simulink model "HEV_Simu_V1_1_VectVir"  (R2018a)
settings: Solver=ode23s  StartTime=0.0  StopTime=660  FixedStep=0.001  EnableMultiTasking=on
PreLoadFcn:
  | HevSimuVccWs_V1_PreLoad
StartFcn:
  | tic
StopFcn:
  | toc
  | disp(['実時間の' num2str(max(tout)/toc) '倍速'])
model workspace (MAT data in the model file):
  Var = 0
undefined symbols (not defined in the file or in its folder): canChannel
libraries: canmsglib x55, canlib x35, simulink x2, sldrtlib x1
(part 4 of 4)

== system HEV_Simu_V1_1_VectVir/Controller/CtrlStrct_VNT_Level_2/VNT_Level_2_CAN/Gateway/Gateway PwtrCAN/Gateway_VehCAN_Receive_50ms ==
  VehCAN_Msg : Inport
  function : TriggerPort  TriggerType=function-call  VariantControl=Variant
  Gateway_VehCAN Unpack2 : canmsglib/CAN Unpack  CANdbFile=HEV_CANDB.dbc  MsgList=BodyCtrl_VehCAN_Tx  MsgName=BodyCtrl_VehCAN_Tx  MsgIDType=Extended (29-bit identifier)  MsgIdentifier=218079272  MsgLength=8  SignalInfo=BdyCtrl_Door_open_flag$1$1$1$2$1$0$1$0$0$1$#BdyCtrl_Engine_hood_open_flag$1$1$1$2$1$0$1$0$0$1$#BdyCtrl_Idlestop_cancel$0$1$1$2$1$0$1$0$0$1$#  NSignals=3  IDPort=off  TimestampPort=off  ErrorPort=off  RemotePort=off  LengthPort=off  StatusPort=off  StartBits=str2num('[int32(1);int32(1);int32(0)]')  SignalSizes=str2num('[int32(1);int32(1);int32(1)]')  ByteOrders=str2num('[int32(1);int32(1);int32(1)]')  DataTypes=str2num('[int32(2);int32(2);int32(2)]')  MultiplexTypes=str2num('[int32(1);int32(1);int32(1)]')  MultiplexValues=str2num('[double(0);double(0);double(0)]')  Factors=str2num('[double(1);double(1);double(1)]')  Offsets=str2num('[double(0);double(0);double(0)]')  Minimums=str2num('[double(0);double(0);double(0)]')  Maximums=str2num('[double(1);double(1);double(1)]')  ApplyMinMax=off
      settings: AttributesFormatString=<CANdbFile = %<CANdbFile>>  SourceProductName=Simulink Real-Time  SourceProductBaseCode=XP  DataFormat=CANdb specified signals
  Gateway_VehCAN Unpack4 : canmsglib/CAN Unpack  CANdbFile=HEV_CANDB.dbc  MsgList=HVAC_Ctrl_VehCAN_Tx  MsgName=HVAC_Ctrl_VehCAN_Tx  MsgIDType=Extended (29-bit identifier)  MsgIdentifier=218095751  MsgLength=8  SignalInfo=HVAC_Ctrl_Idlestop_cancel$1$1$1$2$1$0$1$0$0$1$#HVAC_Ctrl_Idlestop_enbl$0$1$1$2$1$0$1$0$0$1$#  NSignals=2  IDPort=off  TimestampPort=off  ErrorPort=off  RemotePort=off  LengthPort=off  StatusPort=off  StartBits=str2num('[int32(1);int32(0)]')  SignalSizes=str2num('[int32(1);int32(1)]')  ByteOrders=str2num('[int32(1);int32(1)]')  DataTypes=str2num('[int32(2);int32(2)]')  MultiplexTypes=str2num('[int32(1);int32(1)]')  MultiplexValues=str2num('[double(0);double(0)]')  Factors=str2num('[double(1);double(1)]')  Offsets=str2num('[double(0);double(0)]')  Minimums=str2num('[double(0);double(0)]')  Maximums=str2num('[double(1);double(1)]')  ApplyMinMax=off
      settings: AttributesFormatString=<CANdbFile = %<CANdbFile>>  SourceProductName=Simulink Real-Time  SourceProductBaseCode=XP  DataFormat=CANdb specified signals
  Gateway_VehCAN Unpack5 : canmsglib/CAN Unpack  CANdbFile=HEV_CANDB.dbc  MsgList=SteerCtrl_VehCAN_Tx  MsgName=SteerCtrl_VehCAN_Tx  MsgIDType=Extended (29-bit identifier)  MsgIdentifier=218066963  MsgLength=8  SignalInfo=StrgCtrl_Steer_angle$0$16$1$1$1$0$3.125000e-02$0$-720$720$#  NSignals=1  IDPort=off  TimestampPort=off  ErrorPort=off  RemotePort=off  LengthPort=off  StatusPort=off  StartBits=str2num('[int32(0)]')  SignalSizes=str2num('[int32(16)]')  ByteOrders=str2num('[int32(1)]')  DataTypes=str2num('[int32(1)]')  MultiplexTypes=str2num('[int32(1)]')  MultiplexValues=str2num('[double(0)]')  Factors=str2num('[double(3.125000e-02)]')  Offsets=str2num('[double(0)]')  Minimums=str2num('[double(-720)]')  Maximums=str2num('[double(720)]')  ApplyMinMax=off
      settings: AttributesFormatString=<CANdbFile = %<CANdbFile>>  SourceProductName=Simulink Real-Time  SourceProductBaseCode=XP  DataFormat=CANdb specified signals
  BdyCtrl_Door_open_flag : Outport
  BdyCtrl_Engine_hood_open_flag : Outport  Port=2
  BdyCtrl_Idlestop_cancel : Outport  Port=3
  HVAC_Ctrl_Idlestop_cancel : Outport  Port=4
  HVAC_Ctrl_Idlestop_enbl : Outport  Port=5
  StrgCtrl_Steer_angle : Outport  Port=6
  wires:
  Gateway_VehCAN Unpack5/1 -> StrgCtrl_Steer_angle/1  "VehCAN_StrgCtrl_Steer_angle"
  VehCAN_Msg/1 -> Gateway_VehCAN Unpack5/1, Gateway_VehCAN Unpack4/1, Gateway_VehCAN Unpack2/1
  Gateway_VehCAN Unpack4/1 -> HVAC_Ctrl_Idlestop_cancel/1  "VehCAN_HVAC_Ctrl_Idlestop_cancel"
  Gateway_VehCAN Unpack4/2 -> HVAC_Ctrl_Idlestop_enbl/1  "VehCAN_HVAC_Ctrl_Idlestop_enbl"
  Gateway_VehCAN Unpack2/1 -> BdyCtrl_Door_open_flag/1  "VehCAN_BdyCtrl_Door_open_flag"
  Gateway_VehCAN Unpack2/3 -> BdyCtrl_Idlestop_cancel/1  "VehCAN_BdyCtrl_Idlestop_cancel"
  Gateway_VehCAN Unpack2/2 -> BdyCtrl_Engine_hood_open_flag/1  "VehCAN_BdyCtrl_Engine_hood_open_flag"

== system HEV_Simu_V1_1_VectVir/Controller/CtrlStrct_VNT_Level_2/VNT_Level_2_CAN/Gateway/Gateway VehCAN/Gateway_InfoCAN_Receive_100ms ==
  InfoCAN_Msg : Inport
  function : TriggerPort  TriggerType=function-call  VariantControl=Variant
  Radar_InfoCAN Unpack : canmsglib/CAN Unpack  CANdbFile=HEV_CANDB.dbc  MsgList=Radar_InfoCAN_Tx  MsgName=Radar_InfoCAN_Tx  MsgIDType=Extended (29-bit identifier)  MsgIdentifier=218038400  MsgLength=8  SignalInfo=Radar_Relative_distance$0$16$1$2$1$0$1.000000e-02$0$0$500$#Radar_Relative_velocity$16$16$1$1$1$0$1.000000e-02$0$-50$50$#  NSignals=2  IDPort=off  TimestampPort=off  ErrorPort=off  RemotePort=off  LengthPort=off  StatusPort=off  StartBits=str2num('[int32(0);int32(16)]')  SignalSizes=str2num('[int32(16);int32(16)]')  ByteOrders=str2num('[int32(1);int32(1)]')  DataTypes=str2num('[int32(2);int32(1)]')  MultiplexTypes=str2num('[int32(1);int32(1)]')  MultiplexValues=str2num('[double(0);double(0)]')  Factors=str2num('[double(1.000000e-02);double(1.000000e-02)]')  Offsets=str2num('[double(0);double(0)]')  Minimums=str2num('[double(0);double(-50)]')  Maximums=str2num('[double(500);double(50)]')  ApplyMinMax=off
      settings: AttributesFormatString=<CANdbFile = %<CANdbFile>>  SourceProductName=Simulink Real-Time  SourceProductBaseCode=XP  DataFormat=CANdb specified signals
  Radar_Relative_distance : Outport
  Radar_Relative_velocity : Outport  Port=2
  wires:
  Radar_InfoCAN Unpack/2 -> Radar_Relative_velocity/1  "InfoCAN_Radar_Relative_velocity"
  InfoCAN_Msg/1 -> Radar_InfoCAN Unpack/1
  Radar_InfoCAN Unpack/1 -> Radar_Relative_distance/1  "InfoCAN_Radar_Relative_distance"

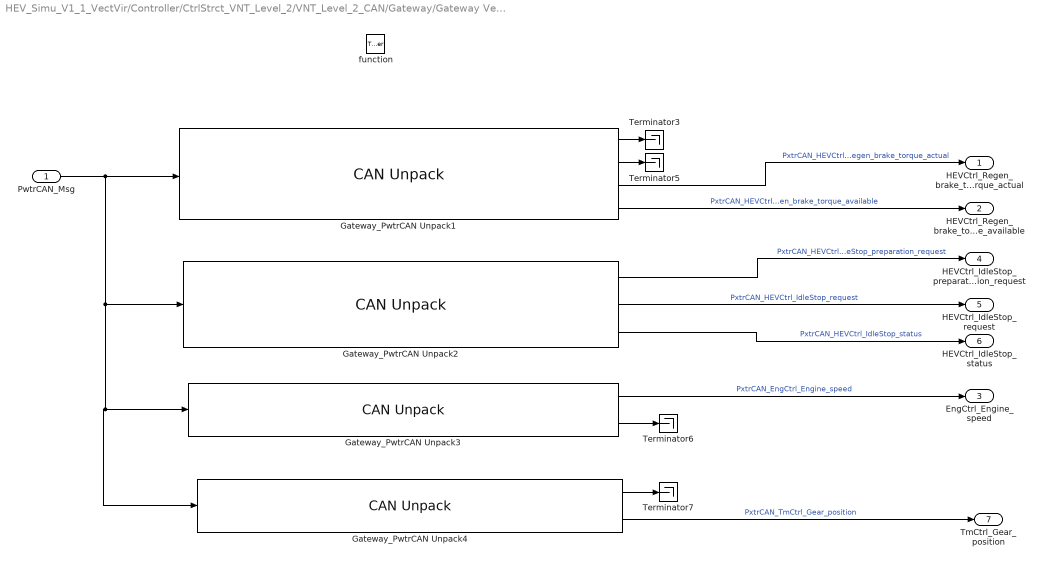
== system HEV_Simu_V1_1_VectVir/Controller/CtrlStrct_VNT_Level_2/VNT_Level_2_CAN/Gateway/Gateway VehCAN/Gateway_PwtrCAN_Receive_10ms ==
  PwtrCAN_Msg : Inport
  function : TriggerPort  TriggerType=function-call  VariantControl=Variant
  Gateway_PwtrCAN Unpack1 : canmsglib/CAN Unpack  CANdbFile=HEV_CANDB.dbc  MsgList=HEV_Ctrl_PwtrCAN_Tx_1  MsgName=HEV_Ctrl_PwtrCAN_Tx_1  MsgIDType=Extended (29-bit identifier)  MsgIdentifier=218046594  MsgLength=8  SignalInfo=HEVCtrl_Engine_torque_request$0$16$1$1$1$0$1.562500e-02$0$-300$300$#HEVCtrl_Motor_torque_request$16$16$1$1$1$0$1.562500e-02$0$-300$300$#HEVCtrl_Regen_brake_torque_actua$48$16$1$1$1$0$6.250000e-02$0$-300$3000$#HEVCtrl_Regen_brake_torque_avail$32$16$1$1$1$0$6.250000e-02$0$-300$3000$#  NSignals=4  IDPort=off  TimestampPort=off  ErrorPort=off  RemotePort=off  LengthPort=off  StatusPort=off  StartBits=str2num('[int32(0);int32(16);int32(48);int32(32)]')  SignalSizes=str2num('[int32(16);int32(16);int32(16);int32(16)]')  ByteOrders=str2num('[int32(1);int32(1);int32(1);int32(1)]')  DataTypes=str2num('[int32(1);int32(1);int32(1);int32(1)]')  MultiplexTypes=str2num('[int32(1);int32(1);int32(1);int32(1)]')  MultiplexValues=str2num('[double(0);double(0);double(0);double(0)]')  Factors=str2num('[double(1.562500e-02);double(1.562500e-02);double(6.250000e-02);double(6.250000e-02)]')  Offsets=str2num('[double(0);double(0);double(0);double(0)]')  Minimums=str2num('[double(-300);double(-300);double(-300);double(-300)]')  Maximums=str2num('[double(300);double(300);double(3000);double(3000)]')  ApplyMinMax=off
      settings: AttributesFormatString=<CANdbFile = %<CANdbFile>>  SourceProductName=Simulink Real-Time  SourceProductBaseCode=XP  DataFormat=CANdb specified signals
  Gateway_PwtrCAN Unpack2 : canmsglib/CAN Unpack  CANdbFile=HEV_CANDB.dbc  MsgList=HEV_Ctrl_PwtrCAN_Tx_2  MsgName=HEV_Ctrl_PwtrCAN_Tx_2  MsgIDType=Extended (29-bit identifier)  MsgIdentifier=218046850  MsgLength=8  SignalInfo=HEV_IdleStopCtrl_preparation_req$0$1$1$2$1$0$1$0$0$1$#HEV_IdleStopCtrl_request$1$1$1$2$1$0$1$0$0$1$#HEV_IdleStopCtrl_status$2$1$1$2$1$0$1$0$0$1$#  NSignals=3  IDPort=off  TimestampPort=off  ErrorPort=off  RemotePort=off  LengthPort=off  StatusPort=off  StartBits=str2num('[int32(0);int32(1);int32(2)]')  SignalSizes=str2num('[int32(1);int32(1);int32(1)]')  ByteOrders=str2num('[int32(1);int32(1);int32(1)]')  DataTypes=str2num('[int32(2);int32(2);int32(2)]')  MultiplexTypes=str2num('[int32(1);int32(1);int32(1)]')  MultiplexValues=str2num('[double(0);double(0);double(0)]')  Factors=str2num('[double(1);double(1);double(1)]')  Offsets=str2num('[double(0);double(0);double(0)]')  Minimums=str2num('[double(0);double(0);double(0)]')  Maximums=str2num('[double(1);double(1);double(1)]')  ApplyMinMax=off
      settings: AttributesFormatString=<CANdbFile = %<CANdbFile>>  SourceProductName=Simulink Real-Time  SourceProductBaseCode=XP  DataFormat=CANdb specified signals
  Gateway_PwtrCAN Unpack3 : canmsglib/CAN Unpack  CANdbFile=HEV_CANDB.dbc  MsgList=EngineCtrl_PwtrCAN_Tx  MsgName=EngineCtrl_PwtrCAN_Tx  MsgIDType=Extended (29-bit identifier)  MsgIdentifier=218050560  MsgLength=8  SignalInfo=EngCtrl_Engine_speed$0$16$1$2$1$0$1.250000e-01$0$0$8192$#EngCtrl_Engine_torque_actual$16$16$1$1$1$0$1.562500e-02$0$-300$300$#  NSignals=2  IDPort=off  TimestampPort=off  ErrorPort=off  RemotePort=off  LengthPort=off  StatusPort=off  StartBits=str2num('[int32(0);int32(16)]')  SignalSizes=str2num('[int32(16);int32(16)]')  ByteOrders=str2num('[int32(1);int32(1)]')  DataTypes=str2num('[int32(2);int32(1)]')  MultiplexTypes=str2num('[int32(1);int32(1)]')  MultiplexValues=str2num('[double(0);double(0)]')  Factors=str2num('[double(1.250000e-01);double(1.562500e-02)]')  Offsets=str2num('[double(0);double(0)]')  Minimums=str2num('[double(0);double(-300)]')  Maximums=str2num('[double(8192);double(300)]')  ApplyMinMax=off
      settings: AttributesFormatString=<CANdbFile = %<CANdbFile>>  SourceProductName=Simulink Real-Time  SourceProductBaseCode=XP  DataFormat=CANdb specified signals
  Gateway_PwtrCAN Unpack4 : canmsglib/CAN Unpack  CANdbFile=HEV_CANDB.dbc  MsgList=TransmCtrl_PwtrCAN_Tx  MsgName=TransmCtrl_PwtrCAN_Tx  MsgIDType=Extended (29-bit identifier)  MsgIdentifier=218054659  MsgLength=8  SignalInfo=TmCtrl_Clutch_position$0$8$1$2$1$0$1.000000e-02$0$0$1$#TmCtrl_Gear_position$8$8$1$2$1$0$1$0$0$5$#  NSignals=2  IDPort=off  TimestampPort=off  ErrorPort=off  RemotePort=off  LengthPort=off  StatusPort=off  StartBits=str2num('[int32(0);int32(8)]')  SignalSizes=str2num('[int32(8);int32(8)]')  ByteOrders=str2num('[int32(1);int32(1)]')  DataTypes=str2num('[int32(2);int32(2)]')  MultiplexTypes=str2num('[int32(1);int32(1)]')  MultiplexValues=str2num('[double(0);double(0)]')  Factors=str2num('[double(1.000000e-02);double(1)]')  Offsets=str2num('[double(0);double(0)]')  Minimums=str2num('[double(0);double(0)]')  Maximums=str2num('[double(1);double(5)]')  ApplyMinMax=off
      settings: AttributesFormatString=<CANdbFile = %<CANdbFile>>  SourceProductName=Simulink Real-Time  SourceProductBaseCode=XP  DataFormat=CANdb specified signals
  Terminator{3,5..7} (4 alike) : Terminator
  HEVCtrl_Regen_brake_torque_actual : Outport
  HEVCtrl_Regen_brake_torque_available : Outport  Port=2
  EngCtrl_Engine_speed : Outport  Port=3
  HEVCtrl_IdleStop_preparation_request : Outport  Port=4
  HEVCtrl_IdleStop_request : Outport  Port=5
  HEVCtrl_IdleStop_status : Outport  Port=6
  TmCtrl_Gear_position : Outport  Port=7
  wires:
  Gateway_PwtrCAN Unpack1/4 -> HEVCtrl_Regen_brake_torque_available/1  "PxtrCAN_HEVCtrl_Regen_brake_torque_available"
  Gateway_PwtrCAN Unpack2/1 -> HEVCtrl_IdleStop_preparation_request/1  "PxtrCAN_HEVCtrl_IdleStop_preparation_request"
  Gateway_PwtrCAN Unpack3/1 -> EngCtrl_Engine_speed/1  "PxtrCAN_EngCtrl_Engine_speed"
  Gateway_PwtrCAN Unpack3/2 -> Terminator6/1
  Gateway_PwtrCAN Unpack1/2 -> Terminator5/1
  Gateway_PwtrCAN Unpack1/1 -> Terminator3/1
  Gateway_PwtrCAN Unpack4/2 -> TmCtrl_Gear_position/1  "PxtrCAN_TmCtrl_Gear_position"
  PwtrCAN_Msg/1 -> Gateway_PwtrCAN Unpack1/1, Gateway_PwtrCAN Unpack3/1, Gateway_PwtrCAN Unpack4/1, Gateway_PwtrCAN Unpack2/1
  Gateway_PwtrCAN Unpack2/2 -> HEVCtrl_IdleStop_request/1  "PxtrCAN_HEVCtrl_IdleStop_request"
  Gateway_PwtrCAN Unpack4/1 -> Terminator7/1
  Gateway_PwtrCAN Unpack1/3 -> HEVCtrl_Regen_brake_torque_actual/1  "PxtrCAN_HEVCtrl_Regen_brake_torque_actual"
  Gateway_PwtrCAN Unpack2/3 -> HEVCtrl_IdleStop_status/1  "PxtrCAN_HEVCtrl_IdleStop_status"

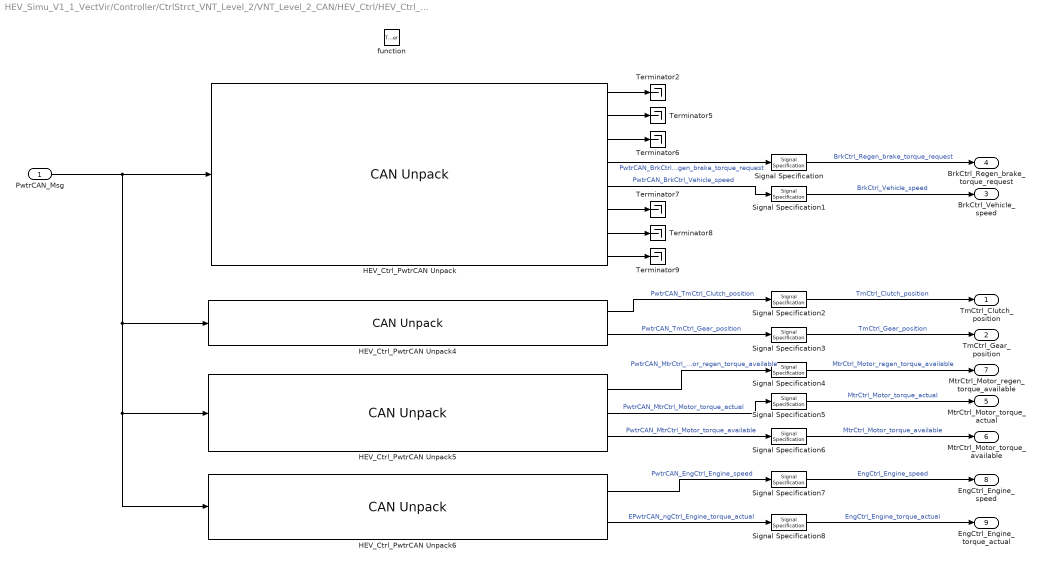
== system HEV_Simu_V1_1_VectVir/Controller/CtrlStrct_VNT_Level_2/VNT_Level_2_CAN/HEV_Ctrl/HEV_Ctrl_PwtrCAN_Rx/HEV_Ctrl_PwtrCAN_Receive_10ms ==
  PwtrCAN_Msg : Inport
  function : TriggerPort  TriggerType=function-call  VariantControl=Variant
  HEV_Ctrl_PwtrCAN Unpack : canmsglib/CAN Unpack  CANdbFile=HEV_CANDB.dbc  MsgList=Gateway_PwtrCAN_Tx_2  MsgName=Gateway_PwtrCAN_Tx_2  MsgIDType=Extended (29-bit identifier)  MsgIdentifier=218088325  MsgLength=8  SignalInfo=BdyCtrl_Door_open_flag_G$60$1$1$2$1$0$1$0$0$1$#BdyCtrl_Engine_hood_open_flg_G$59$1$1$2$1$0$1$0$0$1$#BdyCtrl_Idlestop_cancel_G$58$1$1$2$1$0$1$0$0$1$#BrkCtrl_Regen_brake_torque_re_G$16$16$1$1$1$0$1.000000e-02$0$-300$300$#BrkCtrl_Vehicle_speed_G$0$16$1$2$1$0$1.000000e-01$0$0$180$#HVAC_Ctrl_Idlestop_cancel_G$57$1$1$2$1$0$1$0$0$1$#HVAC_Ctrl_Idlestop_enbl_G$56$1$1$2$1$0$1$0$0$1$#StrgCtrl_Steer_angle_G$32$16$1$1$1$0$3.125000e-02$0$-720$720$#  NSignals=8  IDPort=off  TimestampPort=off  ErrorPort=off  RemotePort=off  LengthPort=off  StatusPort=off  StartBits=str2num('[int32(60);int32(59);int32(58);int32(16);int32(0);int32(57);int32(56);int32(32)]')  SignalSizes=str2num('[int32(1);int32(1);int32(1);int32(16);int32(16);int32(1);int32(1);int32(16)]')  ByteOrders=str2num('[int32(1);int32(1);int32(1);int32(1);int32(1);int32(1);int32(1);int32(1)]')  DataTypes=str2num('[int32(2);int32(2);int32(2);int32(1);int32(2);int32(2);int32(2);int32(1)]')  MultiplexTypes=str2num('[int32(1);int32(1);int32(1);int32(1);int32(1);int32(1);int32(1);int32(1)]')  MultiplexValues=str2num('[double(0);double(0);double(0);double(0);double(0);double(0);double(0);double(0)]')  Factors=str2num('[double(1);double(1);double(1);double(1.000000e-02);double(1.000000e-01);double(1);double(1);double(3.125000e-02)]')  Offsets=str2num('[double(0);double(0);double(0);double(0);double(0);double(0);double(0);double(0)]')  Minimums=str2num('[double(0);double(0);double(0);double(-300);double(0);double(0);double(0);double(-720)]')  Maximums=str2num('[double(1);double(1);double(1);double(300);double(180);double(1);double(1);double(720)]')  ApplyMinMax=off
      settings: AttributesFormatString=<CANdbFile = %<CANdbFile>>  SourceProductName=Simulink Real-Time  SourceProductBaseCode=XP  DataFormat=CANdb specified signals
  HEV_Ctrl_PwtrCAN Unpack4 : canmsglib/CAN Unpack  CANdbFile=HEV_CANDB.dbc  MsgList=TransmCtrl_PwtrCAN_Tx  MsgName=TransmCtrl_PwtrCAN_Tx  MsgIDType=Extended (29-bit identifier)  MsgIdentifier=218054659  MsgLength=8  SignalInfo=TmCtrl_Clutch_position$0$8$1$2$1$0$1.000000e-02$0$0$1$#TmCtrl_Gear_position$8$8$1$2$1$0$1$0$0$5$#  NSignals=2  IDPort=off  TimestampPort=off  ErrorPort=off  RemotePort=off  LengthPort=off  StatusPort=off  StartBits=str2num('[int32(0);int32(8)]')  SignalSizes=str2num('[int32(8);int32(8)]')  ByteOrders=str2num('[int32(1);int32(1)]')  DataTypes=str2num('[int32(2);int32(2)]')  MultiplexTypes=str2num('[int32(1);int32(1)]')  MultiplexValues=str2num('[double(0);double(0)]')  Factors=str2num('[double(1.000000e-02);double(1)]')  Offsets=str2num('[double(0);double(0)]')  Minimums=str2num('[double(0);double(0)]')  Maximums=str2num('[double(1);double(5)]')  ApplyMinMax=off
      settings: AttributesFormatString=<CANdbFile = %<CANdbFile>>  SourceProductName=Simulink Real-Time  SourceProductBaseCode=XP  DataFormat=CANdb specified signals
  HEV_Ctrl_PwtrCAN Unpack5 : canmsglib/CAN Unpack  CANdbFile=HEV_CANDB.dbc  MsgList=MotorCtrl_PwtrCAN_Tx  MsgName=MotorCtrl_PwtrCAN_Tx  MsgIDType=Extended (29-bit identifier)  MsgIdentifier=218058883  MsgLength=8  SignalInfo=MtrCtrl_Motor_regen_torque_avail$32$16$1$1$1$0$1.000000e-02$0$-300$300$#MtrCtrl_Motor_torque_actual$0$16$1$1$1$0$1.000000e-02$0$-300$300$#MtrCtrl_Motor_torque_available$16$16$1$1$1$0$1.000000e-02$0$-300$300$#  NSignals=3  IDPort=off  TimestampPort=off  ErrorPort=off  RemotePort=off  LengthPort=off  StatusPort=off  StartBits=str2num('[int32(32);int32(0);int32(16)]')  SignalSizes=str2num('[int32(16);int32(16);int32(16)]')  ByteOrders=str2num('[int32(1);int32(1);int32(1)]')  DataTypes=str2num('[int32(1);int32(1);int32(1)]')  MultiplexTypes=str2num('[int32(1);int32(1);int32(1)]')  MultiplexValues=str2num('[double(0);double(0);double(0)]')  Factors=str2num('[double(1.000000e-02);double(1.000000e-02);double(1.000000e-02)]')  Offsets=str2num('[double(0);double(0);double(0)]')  Minimums=str2num('[double(-300);double(-300);double(-300)]')  Maximums=str2num('[double(300);double(300);double(300)]')  ApplyMinMax=off
      settings: AttributesFormatString=<CANdbFile = %<CANdbFile>>  SourceProductName=Simulink Real-Time  SourceProductBaseCode=XP  DataFormat=CANdb specified signals
  HEV_Ctrl_PwtrCAN Unpack6 : canmsglib/CAN Unpack  CANdbFile=HEV_CANDB.dbc  MsgList=EngineCtrl_PwtrCAN_Tx  MsgName=EngineCtrl_PwtrCAN_Tx  MsgIDType=Extended (29-bit identifier)  MsgIdentifier=218050560  MsgLength=8  SignalInfo=EngCtrl_Engine_speed$0$16$1$2$1$0$1.250000e-01$0$0$8192$#EngCtrl_Engine_torque_actual$16$16$1$1$1$0$1.562500e-02$0$-300$300$#  NSignals=2  IDPort=off  TimestampPort=off  ErrorPort=off  RemotePort=off  LengthPort=off  StatusPort=off  StartBits=str2num('[int32(0);int32(16)]')  SignalSizes=str2num('[int32(16);int32(16)]')  ByteOrders=str2num('[int32(1);int32(1)]')  DataTypes=str2num('[int32(2);int32(1)]')  MultiplexTypes=str2num('[int32(1);int32(1)]')  MultiplexValues=str2num('[double(0);double(0)]')  Factors=str2num('[double(1.250000e-01);double(1.562500e-02)]')  Offsets=str2num('[double(0);double(0)]')  Minimums=str2num('[double(0);double(-300)]')  Maximums=str2num('[double(8192);double(300)]')  ApplyMinMax=off
      settings: AttributesFormatString=<CANdbFile = %<CANdbFile>>  SourceProductName=Simulink Real-Time  SourceProductBaseCode=XP  DataFormat=CANdb specified signals
  Signal Specification{,1..8} (9 alike) : SignalSpecification
  Terminator{2,5..9} (6 alike) : Terminator
  TmCtrl_Clutch_position : Outport
  TmCtrl_Gear_position : Outport  Port=2
  BrkCtrl_Vehicle_speed : Outport  Port=3
  BrkCtrl_Regen_brake_torque_request : Outport  Port=4
  MtrCtrl_Motor_torque_actual : Outport  Port=5
  MtrCtrl_Motor_torque_available : Outport  Port=6
  MtrCtrl_Motor_regen_torque_available : Outport  Port=7
  EngCtrl_Engine_speed : Outport  Port=8
  EngCtrl_Engine_torque_actual : Outport  Port=9
  wires:
  HEV_Ctrl_PwtrCAN Unpack/1 -> Terminator2/1
  PwtrCAN_Msg/1 -> HEV_Ctrl_PwtrCAN Unpack4/1, HEV_Ctrl_PwtrCAN Unpack5/1, HEV_Ctrl_PwtrCAN Unpack6/1, HEV_Ctrl_PwtrCAN Unpack/1
  HEV_Ctrl_PwtrCAN Unpack/6 -> Terminator7/1
  HEV_Ctrl_PwtrCAN Unpack/3 -> Terminator6/1
  HEV_Ctrl_PwtrCAN Unpack/8 -> Terminator9/1
  HEV_Ctrl_PwtrCAN Unpack/5 -> Signal Specification1/1  "PwtrCAN_BrkCtrl_Vehicle_speed"
  HEV_Ctrl_PwtrCAN Unpack6/2 -> Signal Specification8/1  "EPwtrCAN_ngCtrl_Engine_torque_actual"
  HEV_Ctrl_PwtrCAN Unpack/2 -> Terminator5/1
  HEV_Ctrl_PwtrCAN Unpack/7 -> Terminator8/1
  HEV_Ctrl_PwtrCAN Unpack5/1 -> Signal Specification4/1  "PwtrCAN_MtrCtrl_Motor_regen_torque_available"
  HEV_Ctrl_PwtrCAN Unpack6/1 -> Signal Specification7/1  "PwtrCAN_EngCtrl_Engine_speed"
  HEV_Ctrl_PwtrCAN Unpack5/2 -> Signal Specification5/1  "PwtrCAN_MtrCtrl_Motor_torque_actual"
  HEV_Ctrl_PwtrCAN Unpack/4 -> Signal Specification/1  "PwtrCAN_BrkCtrl_Regen_brake_torque_request"
  HEV_Ctrl_PwtrCAN Unpack5/3 -> Signal Specification6/1  "PwtrCAN_MtrCtrl_Motor_torque_available"
  HEV_Ctrl_PwtrCAN Unpack4/1 -> Signal Specification2/1  "PwtrCAN_TmCtrl_Clutch_position"
  HEV_Ctrl_PwtrCAN Unpack4/2 -> Signal Specification3/1  "PwtrCAN_TmCtrl_Gear_position"
  Signal Specification/1 -> BrkCtrl_Regen_brake_torque_request/1  "BrkCtrl_Regen_brake_torque_request"
  Signal Specification1/1 -> BrkCtrl_Vehicle_speed/1  "BrkCtrl_Vehicle_speed"
  Signal Specification2/1 -> TmCtrl_Clutch_position/1  "TmCtrl_Clutch_position"
  Signal Specification3/1 -> TmCtrl_Gear_position/1  "TmCtrl_Gear_position"
  Signal Specification4/1 -> MtrCtrl_Motor_regen_torque_available/1  "MtrCtrl_Motor_regen_torque_available"
  Signal Specification5/1 -> MtrCtrl_Motor_torque_actual/1  "MtrCtrl_Motor_torque_actual"
  Signal Specification6/1 -> MtrCtrl_Motor_torque_available/1  "MtrCtrl_Motor_torque_available"
  Signal Specification7/1 -> EngCtrl_Engine_speed/1  "EngCtrl_Engine_speed"
  Signal Specification8/1 -> EngCtrl_Engine_torque_actual/1  "EngCtrl_Engine_torque_actual"

== system HEV_Simu_V1_1_VectVir/Controller/CtrlStrct_VNT_Level_2/VNT_Level_2_CAN/HEV_Ctrl/HEV_Ctrl_PwtrCAN_Rx/HEV_Ctrl_PwtrCAN_Receive_50ms ==
  PwtrCAN_Msg : Inport
  function : TriggerPort  TriggerType=function-call  VariantControl=Variant
  HEV_Ctrl_PwtrCAN Unpack2 : canmsglib/CAN Unpack  CANdbFile=HEV_CANDB.dbc  MsgList=Gateway_PwtrCAN_Tx_1  MsgName=Gateway_PwtrCAN_Tx_1  MsgIDType=Extended (29-bit identifier)  MsgIdentifier=218088069  MsgLength=8  SignalInfo=NAVI_Home_around_status_G$0$16$1$2$1$0$1$0$0$65535$#VMCtrl_PropTorqCmnd_G$24$16$1$1$1$0$1.000000e-02$0$-300$300$#VMCtrl_PropTorqStatus_G$16$8$1$2$1$0$1$0$0$7$#  NSignals=3  IDPort=off  TimestampPort=off  ErrorPort=off  RemotePort=off  LengthPort=off  StatusPort=off  StartBits=str2num('[int32(0);int32(24);int32(16)]')  SignalSizes=str2num('[int32(16);int32(16);int32(8)]')  ByteOrders=str2num('[int32(1);int32(1);int32(1)]')  DataTypes=str2num('[int32(2);int32(1);int32(2)]')  MultiplexTypes=str2num('[int32(1);int32(1);int32(1)]')  MultiplexValues=str2num('[double(0);double(0);double(0)]')  Factors=str2num('[double(1);double(1.000000e-02);double(1)]')  Offsets=str2num('[double(0);double(0);double(0)]')  Minimums=str2num('[double(0);double(-300);double(0)]')  Maximums=str2num('[double(65535);double(300);double(7)]')  ApplyMinMax=off
      settings: AttributesFormatString=<CANdbFile = %<CANdbFile>>  SourceProductName=Simulink Real-Time  SourceProductBaseCode=XP  DataFormat=CANdb specified signals
  HEV_Ctrl_PwtrCAN Unpack3 : canmsglib/CAN Unpack  CANdbFile=HEV_CANDB.dbc  MsgList=BatteryCtrl_PwtrCAN_Tx  MsgName=BatteryCtrl_PwtrCAN_Tx  MsgIDType=Extended (29-bit identifier)  MsgIdentifier=218071172  MsgLength=8  SignalInfo=BatCtrl_SOC$0$16$1$2$1$0$3.906250e-03$0$0$100$#  NSignals=1  IDPort=off  TimestampPort=off  ErrorPort=off  RemotePort=off  LengthPort=off  StatusPort=off  StartBits=str2num('[int32(0)]')  SignalSizes=str2num('[int32(16)]')  ByteOrders=str2num('[int32(1)]')  DataTypes=str2num('[int32(2)]')  MultiplexTypes=str2num('[int32(1)]')  MultiplexValues=str2num('[double(0)]')  Factors=str2num('[double(3.906250e-03)]')  Offsets=str2num('[double(0)]')  Minimums=str2num('[double(0)]')  Maximums=str2num('[double(100)]')  ApplyMinMax=off
      settings: AttributesFormatString=<CANdbFile = %<CANdbFile>>  SourceProductName=Simulink Real-Time  SourceProductBaseCode=XP  DataFormat=CANdb specified signals
  Signal Specification{,1..3} (4 alike) : SignalSpecification
  BatCtrl_SOC : Outport
  VMCtrl_PropTorqStatus : Outport  Port=2
  VMCtrl_PropTorqCmnd : Outport  Port=3
  NAVI_Home_around_status : Outport  Port=4
  wires:
  HEV_Ctrl_PwtrCAN Unpack2/1 -> Signal Specification/1  "PwtrCAN_NAVI_Home_around_status"
  PwtrCAN_Msg/1 -> HEV_Ctrl_PwtrCAN Unpack3/1, HEV_Ctrl_PwtrCAN Unpack2/1
  HEV_Ctrl_PwtrCAN Unpack3/1 -> Signal Specification3/1  "PwtrCAN_BatCtrl_SOC"
  HEV_Ctrl_PwtrCAN Unpack2/2 -> Signal Specification1/1  "PwtrCAN_VMCtrl_PropTorqCmnd"
  HEV_Ctrl_PwtrCAN Unpack2/3 -> Signal Specification2/1  "PwtrCAN_VMCtrl_PropTorqStatus"
  Signal Specification/1 -> NAVI_Home_around_status/1  "NAVI_Home_around_status"
  Signal Specification1/1 -> VMCtrl_PropTorqCmnd/1  "VMCtrl_PropTorqCmnd"
  Signal Specification2/1 -> VMCtrl_PropTorqStatus/1  "VMCtrl_PropTorqStatus"
  Signal Specification3/1 -> BatCtrl_SOC/1  "BatCtrl_SOC"

== system HEV_Simu_V1_1_VectVir/Controller/CtrlStrct_VNT_Level_2/VNT_Level_2_CAN/HVAC_Ctrl/HVAC_Ctrl_VehCAN_Rx/HVAC_Ctrl_VehCAN_Receive_50ms ==
  VehCAN_Msg : Inport
  function : TriggerPort  TriggerType=function-call  VariantControl=Variant
  HVAC_Ctrl_VehCAN Unpack : canmsglib/CAN Unpack  CANdbFile=HEV_CANDB.dbc  MsgList=Gateway_VehCAN_Tx_2  MsgName=Gateway_VehCAN_Tx_2  MsgIDType=Extended (29-bit identifier)  MsgIdentifier=218087813  MsgLength=8  SignalInfo=EngCtrl_Engine_speed_G$0$16$1$2$1$0$1.250000e-01$0$0$8192$#HEV_IdleStopCtrl_preparation_r_G$24$1$1$2$1$0$1$0$0$1$#HEV_IdleStopCtrl_request_G$25$1$1$2$1$0$1$0$0$1$#HEV_IdleStopCtrl_status_G$26$1$1$2$1$0$1$0$0$1$#TmCtrl_Gear_position_G$16$8$1$2$1$0$1$0$0$5$#  NSignals=5  IDPort=off  TimestampPort=off  ErrorPort=off  RemotePort=off  LengthPort=off  StatusPort=off  StartBits=str2num('[int32(0);int32(24);int32(25);int32(26);int32(16)]')  SignalSizes=str2num('[int32(16);int32(1);int32(1);int32(1);int32(8)]')  ByteOrders=str2num('[int32(1);int32(1);int32(1);int32(1);int32(1)]')  DataTypes=str2num('[int32(2);int32(2);int32(2);int32(2);int32(2)]')  MultiplexTypes=str2num('[int32(1);int32(1);int32(1);int32(1);int32(1)]')  MultiplexValues=str2num('[double(0);double(0);double(0);double(0);double(0)]')  Factors=str2num('[double(1.250000e-01);double(1);double(1);double(1);double(1)]')  Offsets=str2num('[double(0);double(0);double(0);double(0);double(0)]')  Minimums=str2num('[double(0);double(0);double(0);double(0);double(0)]')  Maximums=str2num('[double(8192);double(1);double(1);double(1);double(5)]')  ApplyMinMax=off
      settings: AttributesFormatString=<CANdbFile = %<CANdbFile>>  SourceProductName=Simulink Real-Time  SourceProductBaseCode=XP  DataFormat=CANdb specified signals
  Signal Specification : SignalSpecification
  Signal Specification1 : SignalSpecification
  Signal Specification2 : SignalSpecification
  Terminator6 : Terminator
  Terminator8 : Terminator
  EngCtrl_Engine_speed : Outport
  HEVCtrl_IdleStop_preparation_request : Outport  Port=2
  HEVCtrl_IdleStop_status : Outport  Port=3
  wires:
  HVAC_Ctrl_VehCAN Unpack/4 -> Signal Specification2/1  "VehCAN_HEVCtrl_IdleStop_status"
  HVAC_Ctrl_VehCAN Unpack/5 -> Terminator8/1
  HVAC_Ctrl_VehCAN Unpack/2 -> Signal Specification/1  "VehCAN_HEVCtrl_IdleStop_preparation_request"
  HVAC_Ctrl_VehCAN Unpack/3 -> Terminator6/1
  HVAC_Ctrl_VehCAN Unpack/1 -> Signal Specification1/1  "VehCAN_EngCtrl_Engine_speed"
  VehCAN_Msg/1 -> HVAC_Ctrl_VehCAN Unpack/1
  Signal Specification/1 -> HEVCtrl_IdleStop_preparation_request/1  "HEVCtrl_IdleStop_preparation_request"
  Signal Specification1/1 -> EngCtrl_Engine_speed/1  "EngCtrl_Engine_speed"
  Signal Specification2/1 -> HEVCtrl_IdleStop_status/1  "HEVCtrl_IdleStop_status"

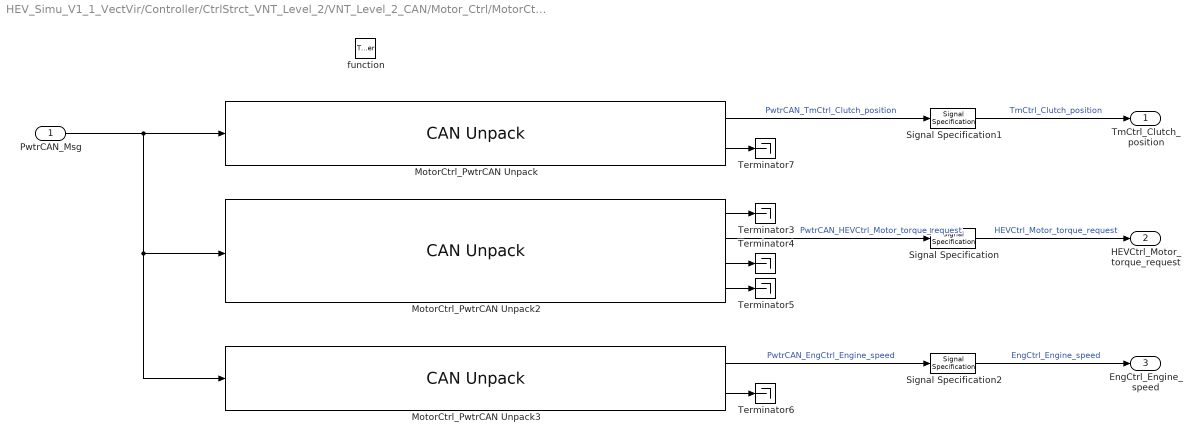
== system HEV_Simu_V1_1_VectVir/Controller/CtrlStrct_VNT_Level_2/VNT_Level_2_CAN/Motor_Ctrl/MotorCtrl_PwtrCAN_Rx/MotorCtrl_PwtrCAN_Receive_10ms ==
  PwtrCAN_Msg : Inport
  function : TriggerPort  TriggerType=function-call  VariantControl=Variant
  MotorCtrl_PwtrCAN Unpack : canmsglib/CAN Unpack  CANdbFile=HEV_CANDB.dbc  MsgList=TransmCtrl_PwtrCAN_Tx  MsgName=TransmCtrl_PwtrCAN_Tx  MsgIDType=Extended (29-bit identifier)  MsgIdentifier=218054659  MsgLength=8  SignalInfo=TmCtrl_Clutch_position$0$8$1$2$1$0$1.000000e-02$0$0$1$#TmCtrl_Gear_position$8$8$1$2$1$0$1$0$0$5$#  NSignals=2  IDPort=off  TimestampPort=off  ErrorPort=off  RemotePort=off  LengthPort=off  StatusPort=off  StartBits=str2num('[int32(0);int32(8)]')  SignalSizes=str2num('[int32(8);int32(8)]')  ByteOrders=str2num('[int32(1);int32(1)]')  DataTypes=str2num('[int32(2);int32(2)]')  MultiplexTypes=str2num('[int32(1);int32(1)]')  MultiplexValues=str2num('[double(0);double(0)]')  Factors=str2num('[double(1.000000e-02);double(1)]')  Offsets=str2num('[double(0);double(0)]')  Minimums=str2num('[double(0);double(0)]')  Maximums=str2num('[double(1);double(5)]')  ApplyMinMax=off
      settings: AttributesFormatString=<CANdbFile = %<CANdbFile>>  SourceProductName=Simulink Real-Time  SourceProductBaseCode=XP  DataFormat=CANdb specified signals
  MotorCtrl_PwtrCAN Unpack2 : canmsglib/CAN Unpack  CANdbFile=HEV_CANDB.dbc  MsgList=HEV_Ctrl_PwtrCAN_Tx_1  MsgName=HEV_Ctrl_PwtrCAN_Tx_1  MsgIDType=Extended (29-bit identifier)  MsgIdentifier=218046594  MsgLength=8  SignalInfo=HEVCtrl_Engine_torque_request$0$16$1$1$1$0$1.562500e-02$0$-300$300$#HEVCtrl_Motor_torque_request$16$16$1$1$1$0$1.562500e-02$0$-300$300$#HEVCtrl_Regen_brake_torque_actua$48$16$1$1$1$0$6.250000e-02$0$-300$3000$#HEVCtrl_Regen_brake_torque_avail$32$16$1$1$1$0$6.250000e-02$0$-300$3000$#  NSignals=4  IDPort=off  TimestampPort=off  ErrorPort=off  RemotePort=off  LengthPort=off  StatusPort=off  StartBits=str2num('[int32(0);int32(16);int32(48);int32(32)]')  SignalSizes=str2num('[int32(16);int32(16);int32(16);int32(16)]')  ByteOrders=str2num('[int32(1);int32(1);int32(1);int32(1)]')  DataTypes=str2num('[int32(1);int32(1);int32(1);int32(1)]')  MultiplexTypes=str2num('[int32(1);int32(1);int32(1);int32(1)]')  MultiplexValues=str2num('[double(0);double(0);double(0);double(0)]')  Factors=str2num('[double(1.562500e-02);double(1.562500e-02);double(6.250000e-02);double(6.250000e-02)]')  Offsets=str2num('[double(0);double(0);double(0);double(0)]')  Minimums=str2num('[double(-300);double(-300);double(-300);double(-300)]')  Maximums=str2num('[double(300);double(300);double(3000);double(3000)]')  ApplyMinMax=off
      settings: AttributesFormatString=<CANdbFile = %<CANdbFile>>  SourceProductName=Simulink Real-Time  SourceProductBaseCode=XP  DataFormat=CANdb specified signals
  MotorCtrl_PwtrCAN Unpack3 : canmsglib/CAN Unpack  CANdbFile=HEV_CANDB.dbc  MsgList=EngineCtrl_PwtrCAN_Tx  MsgName=EngineCtrl_PwtrCAN_Tx  MsgIDType=Extended (29-bit identifier)  MsgIdentifier=218050560  MsgLength=8  SignalInfo=EngCtrl_Engine_speed$0$16$1$2$1$0$1.250000e-01$0$0$8192$#EngCtrl_Engine_torque_actual$16$16$1$1$1$0$1.562500e-02$0$-300$300$#  NSignals=2  IDPort=off  TimestampPort=off  ErrorPort=off  RemotePort=off  LengthPort=off  StatusPort=off  StartBits=str2num('[int32(0);int32(16)]')  SignalSizes=str2num('[int32(16);int32(16)]')  ByteOrders=str2num('[int32(1);int32(1)]')  DataTypes=str2num('[int32(2);int32(1)]')  MultiplexTypes=str2num('[int32(1);int32(1)]')  MultiplexValues=str2num('[double(0);double(0)]')  Factors=str2num('[double(1.250000e-01);double(1.562500e-02)]')  Offsets=str2num('[double(0);double(0)]')  Minimums=str2num('[double(0);double(-300)]')  Maximums=str2num('[double(8192);double(300)]')  ApplyMinMax=off
      settings: AttributesFormatString=<CANdbFile = %<CANdbFile>>  SourceProductName=Simulink Real-Time  SourceProductBaseCode=XP  DataFormat=CANdb specified signals
  Signal Specification : SignalSpecification
  Signal Specification1 : SignalSpecification
  Signal Specification2 : SignalSpecification
  Terminator{3..7} (5 alike) : Terminator
  TmCtrl_Clutch_position : Outport
  HEVCtrl_Motor_torque_request : Outport  Port=2
  EngCtrl_Engine_speed : Outport  Port=3
  wires:
  MotorCtrl_PwtrCAN Unpack2/3 -> Terminator4/1
  MotorCtrl_PwtrCAN Unpack3/2 -> Terminator6/1
  MotorCtrl_PwtrCAN Unpack2/4 -> Terminator5/1
  MotorCtrl_PwtrCAN Unpack2/1 -> Terminator3/1
  MotorCtrl_PwtrCAN Unpack/2 -> Terminator7/1
  PwtrCAN_Msg/1 -> MotorCtrl_PwtrCAN Unpack2/1, MotorCtrl_PwtrCAN Unpack3/1, MotorCtrl_PwtrCAN Unpack/1
  MotorCtrl_PwtrCAN Unpack3/1 -> Signal Specification2/1  "PwtrCAN_EngCtrl_Engine_speed"
  MotorCtrl_PwtrCAN Unpack/1 -> Signal Specification1/1  "PwtrCAN_TmCtrl_Clutch_position"
  MotorCtrl_PwtrCAN Unpack2/2 -> Signal Specification/1  "PwtrCAN_HEVCtrl_Motor_torque_request"
  Signal Specification/1 -> HEVCtrl_Motor_torque_request/1  "HEVCtrl_Motor_torque_request"
  Signal Specification1/1 -> TmCtrl_Clutch_position/1  "TmCtrl_Clutch_position"
  Signal Specification2/1 -> EngCtrl_Engine_speed/1  "EngCtrl_Engine_speed"

== system HEV_Simu_V1_1_VectVir/Controller/CtrlStrct_VNT_Level_2/VNT_Level_2_CAN/NAVI/NAVI_CAN_Rx/NAVI_InfoCAN_Receive_100ms ==
  InfoCAN_Msg : Inport
  function : TriggerPort  TriggerType=function-call  VariantControl=Variant
  NAVI_InfoCAN Unpack : canmsglib/CAN Unpack  CANdbFile=HEV_CANDB.dbc  MsgList=Gateway_InfoCAN_Tx  MsgName=Gateway_InfoCAN_Tx  MsgIDType=Extended (29-bit identifier)  MsgIdentifier=218099848  MsgLength=8  SignalInfo=BrkCtrl_Vehicle_speed_G1$0$16$1$2$1$0$1.000000e-01$0$0$180$#  NSignals=1  IDPort=off  TimestampPort=off  ErrorPort=off  RemotePort=off  LengthPort=off  StatusPort=off  StartBits=str2num('[int32(0)]')  SignalSizes=str2num('[int32(16)]')  ByteOrders=str2num('[int32(1)]')  DataTypes=str2num('[int32(2)]')  MultiplexTypes=str2num('[int32(1)]')  MultiplexValues=str2num('[double(0)]')  Factors=str2num('[double(1.000000e-01)]')  Offsets=str2num('[double(0)]')  Minimums=str2num('[double(0)]')  Maximums=str2num('[double(180)]')  ApplyMinMax=off
      settings: AttributesFormatString=<CANdbFile = %<CANdbFile>>  SourceProductName=Simulink Real-Time  SourceProductBaseCode=XP  DataFormat=CANdb specified signals
  Signal Specification : SignalSpecification
  BrkCtrl_Vehicle_speed : Outport
  wires:
  NAVI_InfoCAN Unpack/1 -> Signal Specification/1  "InfoCAN_BrkCtrl_Vehicle_speed"
  InfoCAN_Msg/1 -> NAVI_InfoCAN Unpack/1
  Signal Specification/1 -> BrkCtrl_Vehicle_speed/1  "BrkCtrl_Vehicle_speed"

== system HEV_Simu_V1_1_VectVir/Controller/CtrlStrct_VNT_Level_2/VNT_Level_2_CAN/Radar/Radar_CAN_Rx/Radar_InfoCAN_Receive_100ms ==
  InfoCAN_Msg : Inport
  function : TriggerPort  TriggerType=function-call  VariantControl=Variant
  Radar_InfoCAN Unpack : canmsglib/CAN Unpack  CANdbFile=HEV_CANDB.dbc  MsgList=Gateway_InfoCAN_Tx  MsgName=Gateway_InfoCAN_Tx  MsgIDType=Extended (29-bit identifier)  MsgIdentifier=218099848  MsgLength=8  SignalInfo=BrkCtrl_Vehicle_speed_G1$0$16$1$2$1$0$1.000000e-01$0$0$180$#  NSignals=1  IDPort=off  TimestampPort=off  ErrorPort=off  RemotePort=off  LengthPort=off  StatusPort=off  StartBits=str2num('[int32(0)]')  SignalSizes=str2num('[int32(16)]')  ByteOrders=str2num('[int32(1)]')  DataTypes=str2num('[int32(2)]')  MultiplexTypes=str2num('[int32(1)]')  MultiplexValues=str2num('[double(0)]')  Factors=str2num('[double(1.000000e-01)]')  Offsets=str2num('[double(0)]')  Minimums=str2num('[double(0)]')  Maximums=str2num('[double(180)]')  ApplyMinMax=off
      settings: AttributesFormatString=<CANdbFile = %<CANdbFile>>  SourceProductName=Simulink Real-Time  SourceProductBaseCode=XP  DataFormat=CANdb specified signals
  Signal Specification : SignalSpecification
  BrkCtrl_Vehicle_speed : Outport
  wires:
  Radar_InfoCAN Unpack/1 -> Signal Specification/1  "InfoCAN_BrkCtrl_Vehicle_speed"
  InfoCAN_Msg/1 -> Radar_InfoCAN Unpack/1
  Signal Specification/1 -> BrkCtrl_Vehicle_speed/1  "BrkCtrl_Vehicle_speed"

== system HEV_Simu_V1_1_VectVir/Controller/CtrlStrct_VNT_Level_2/VNT_Level_2_CAN/Steer_Ctrl/SteerCtrl_VehCAN_Rx/SteerCtrl_VehCAN_Receive50ms ==
  VehCAN_Msg : Inport
  function : TriggerPort  TriggerType=function-call  VariantControl=Variant
  Signal Specification : SignalSpecification
  SteerCtrl_VehCAN Unpack : canmsglib/CAN Unpack  CANdbFile=HEV_CANDB.dbc  MsgList=BrakeCtrl_VehCAN_Tx  MsgName=BrakeCtrl_VehCAN_Tx  MsgIDType=Extended (29-bit identifier)  MsgIdentifier=218062859  MsgLength=8  SignalInfo=BrkCtrl_Regen_brake_torque_reque$16$16$1$1$1$0$1.000000e-02$0$-300$300$#BrkCtrl_Vehicle_speed$0$16$1$2$1$0$1.000000e-01$0$0$180$#  NSignals=2  IDPort=off  TimestampPort=off  ErrorPort=off  RemotePort=off  LengthPort=off  StatusPort=off  StartBits=str2num('[int32(16);int32(0)]')  SignalSizes=str2num('[int32(16);int32(16)]')  ByteOrders=str2num('[int32(1);int32(1)]')  DataTypes=str2num('[int32(1);int32(2)]')  MultiplexTypes=str2num('[int32(1);int32(1)]')  MultiplexValues=str2num('[double(0);double(0)]')  Factors=str2num('[double(1.000000e-02);double(1.000000e-01)]')  Offsets=str2num('[double(0);double(0)]')  Minimums=str2num('[double(-300);double(0)]')  Maximums=str2num('[double(300);double(180)]')  ApplyMinMax=off
      settings: AttributesFormatString=<CANdbFile = %<CANdbFile>>  SourceProductName=Simulink Real-Time  SourceProductBaseCode=XP  DataFormat=CANdb specified signals
  Terminator4 : Terminator
  BrkCtrl_Vehicle_speed : Outport
  wires:
  SteerCtrl_VehCAN Unpack/1 -> Terminator4/1  "VehCAN_BrkCtrl_Regen_brake_torque_request"
  VehCAN_Msg/1 -> SteerCtrl_VehCAN Unpack/1
  SteerCtrl_VehCAN Unpack/2 -> Signal Specification/1  "VehCAN_BrkCtrl_Vehicle_speed"
  Signal Specification/1 -> BrkCtrl_Vehicle_speed/1  "BrkCtrl_Vehicle_speed"

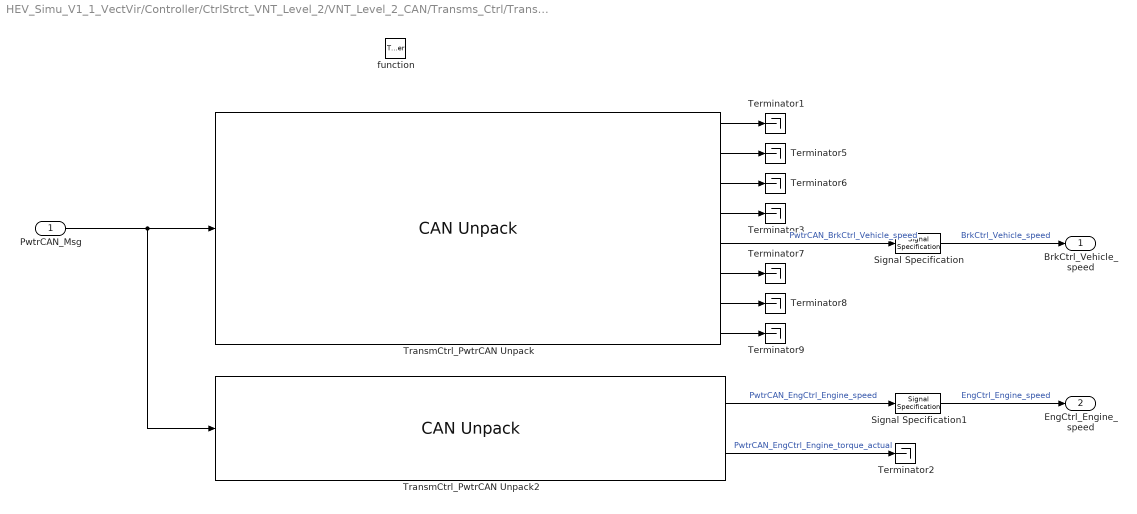
== system HEV_Simu_V1_1_VectVir/Controller/CtrlStrct_VNT_Level_2/VNT_Level_2_CAN/Transms_Ctrl/TransmCtrl_PwtrCAN_Rx/TransmCtrl_PwtrCAN_Receive_10ms ==
  PwtrCAN_Msg : Inport
  function : TriggerPort  TriggerType=function-call  VariantControl=Variant
  Signal Specification : SignalSpecification
  Signal Specification1 : SignalSpecification
  Terminator{1..3,5..9} (8 alike) : Terminator
  TransmCtrl_PwtrCAN Unpack : canmsglib/CAN Unpack  CANdbFile=HEV_CANDB.dbc  MsgList=Gateway_PwtrCAN_Tx_2  MsgName=Gateway_PwtrCAN_Tx_2  MsgIDType=Extended (29-bit identifier)  MsgIdentifier=218088325  MsgLength=8  SignalInfo=BdyCtrl_Door_open_flag_G$60$1$1$2$1$0$1$0$0$1$#BdyCtrl_Engine_hood_open_flg_G$59$1$1$2$1$0$1$0$0$1$#BdyCtrl_Idlestop_cancel_G$58$1$1$2$1$0$1$0$0$1$#BrkCtrl_Regen_brake_torque_re_G$16$16$1$1$1$0$1.000000e-02$0$-300$300$#BrkCtrl_Vehicle_speed_G$0$16$1$2$1$0$1.000000e-01$0$0$180$#HVAC_Ctrl_Idlestop_cancel_G$57$1$1$2$1$0$1$0$0$1$#HVAC_Ctrl_Idlestop_enbl_G$56$1$1$2$1$0$1$0$0$1$#StrgCtrl_Steer_angle_G$32$16$1$1$1$0$3.125000e-02$0$-720$720$#  NSignals=8  IDPort=off  TimestampPort=off  ErrorPort=off  RemotePort=off  LengthPort=off  StatusPort=off  StartBits=str2num('[int32(60);int32(59);int32(58);int32(16);int32(0);int32(57);int32(56);int32(32)]')  SignalSizes=str2num('[int32(1);int32(1);int32(1);int32(16);int32(16);int32(1);int32(1);int32(16)]')  ByteOrders=str2num('[int32(1);int32(1);int32(1);int32(1);int32(1);int32(1);int32(1);int32(1)]')  DataTypes=str2num('[int32(2);int32(2);int32(2);int32(1);int32(2);int32(2);int32(2);int32(1)]')  MultiplexTypes=str2num('[int32(1);int32(1);int32(1);int32(1);int32(1);int32(1);int32(1);int32(1)]')  MultiplexValues=str2num('[double(0);double(0);double(0);double(0);double(0);double(0);double(0);double(0)]')  Factors=str2num('[double(1);double(1);double(1);double(1.000000e-02);double(1.000000e-01);double(1);double(1);double(3.125000e-02)]')  Offsets=str2num('[double(0);double(0);double(0);double(0);double(0);double(0);double(0);double(0)]')  Minimums=str2num('[double(0);double(0);double(0);double(-300);double(0);double(0);double(0);double(-720)]')  Maximums=str2num('[double(1);double(1);double(1);double(300);double(180);double(1);double(1);double(720)]')  ApplyMinMax=off
      settings: AttributesFormatString=<CANdbFile = %<CANdbFile>>  SourceProductName=Simulink Real-Time  SourceProductBaseCode=XP  DataFormat=CANdb specified signals
  TransmCtrl_PwtrCAN Unpack2 : canmsglib/CAN Unpack  CANdbFile=HEV_CANDB.dbc  MsgList=EngineCtrl_PwtrCAN_Tx  MsgName=EngineCtrl_PwtrCAN_Tx  MsgIDType=Extended (29-bit identifier)  MsgIdentifier=218050560  MsgLength=8  SignalInfo=EngCtrl_Engine_speed$0$16$1$2$1$0$1.250000e-01$0$0$8192$#EngCtrl_Engine_torque_actual$16$16$1$1$1$0$1.562500e-02$0$-300$300$#  NSignals=2  IDPort=off  TimestampPort=off  ErrorPort=off  RemotePort=off  LengthPort=off  StatusPort=off  StartBits=str2num('[int32(0);int32(16)]')  SignalSizes=str2num('[int32(16);int32(16)]')  ByteOrders=str2num('[int32(1);int32(1)]')  DataTypes=str2num('[int32(2);int32(1)]')  MultiplexTypes=str2num('[int32(1);int32(1)]')  MultiplexValues=str2num('[double(0);double(0)]')  Factors=str2num('[double(1.250000e-01);double(1.562500e-02)]')  Offsets=str2num('[double(0);double(0)]')  Minimums=str2num('[double(0);double(-300)]')  Maximums=str2num('[double(8192);double(300)]')  ApplyMinMax=off
      settings: AttributesFormatString=<CANdbFile = %<CANdbFile>>  SourceProductName=Simulink Real-Time  SourceProductBaseCode=XP  DataFormat=CANdb specified signals
  BrkCtrl_Vehicle_speed : Outport
  EngCtrl_Engine_speed : Outport  Port=2
  wires:
  TransmCtrl_PwtrCAN Unpack/2 -> Terminator5/1
  TransmCtrl_PwtrCAN Unpack/8 -> Terminator9/1
  TransmCtrl_PwtrCAN Unpack/4 -> Terminator3/1
  TransmCtrl_PwtrCAN Unpack/7 -> Terminator8/1
  TransmCtrl_PwtrCAN Unpack/6 -> Terminator7/1
  TransmCtrl_PwtrCAN Unpack/3 -> Terminator6/1
  TransmCtrl_PwtrCAN Unpack/1 -> Terminator1/1
  TransmCtrl_PwtrCAN Unpack2/2 -> Terminator2/1  "PwtrCAN_EngCtrl_Engine_torque_actual"
  PwtrCAN_Msg/1 -> TransmCtrl_PwtrCAN Unpack2/1, TransmCtrl_PwtrCAN Unpack/1
  TransmCtrl_PwtrCAN Unpack/5 -> Signal Specification/1  "PwtrCAN_BrkCtrl_Vehicle_speed"
  TransmCtrl_PwtrCAN Unpack2/1 -> Signal Specification1/1  "PwtrCAN_EngCtrl_Engine_speed"
  Signal Specification/1 -> BrkCtrl_Vehicle_speed/1  "BrkCtrl_Vehicle_speed"
  Signal Specification1/1 -> EngCtrl_Engine_speed/1  "EngCtrl_Engine_speed"

== system HEV_Simu_V1_1_VectVir/Controller/CtrlStrct_VNT_Level_2/VNT_Level_2_CAN/VM_Ctrl/VM_Ctrl_VehCAN_Rx/VM_Ctrl_VehCAN_Receive_50ms ==
  VehCAN_Msg : Inport
  function : TriggerPort  TriggerType=function-call  VariantControl=Variant
  Signal Specification : SignalSpecification
  Terminator4 : Terminator
  VM_Ctrl_VehCAN Unpack : canmsglib/CAN Unpack  CANdbFile=HEV_CANDB.dbc  MsgList=BrakeCtrl_VehCAN_Tx  MsgName=BrakeCtrl_VehCAN_Tx  MsgIDType=Extended (29-bit identifier)  MsgIdentifier=218062859  MsgLength=8  SignalInfo=BrkCtrl_Regen_brake_torque_reque$16$16$1$1$1$0$1.000000e-02$0$-300$300$#BrkCtrl_Vehicle_speed$0$16$1$2$1$0$1.000000e-01$0$0$180$#  NSignals=2  IDPort=off  TimestampPort=off  ErrorPort=off  RemotePort=off  LengthPort=off  StatusPort=off  StartBits=str2num('[int32(16);int32(0)]')  SignalSizes=str2num('[int32(16);int32(16)]')  ByteOrders=str2num('[int32(1);int32(1)]')  DataTypes=str2num('[int32(1);int32(2)]')  MultiplexTypes=str2num('[int32(1);int32(1)]')  MultiplexValues=str2num('[double(0);double(0)]')  Factors=str2num('[double(1.000000e-02);double(1.000000e-01)]')  Offsets=str2num('[double(0);double(0)]')  Minimums=str2num('[double(-300);double(0)]')  Maximums=str2num('[double(300);double(180)]')  ApplyMinMax=off
      settings: AttributesFormatString=<CANdbFile = %<CANdbFile>>  SourceProductName=Simulink Real-Time  SourceProductBaseCode=XP  DataFormat=CANdb specified signals
  BrkCtrl_Vehicle_speed : Outport
  wires:
  VM_Ctrl_VehCAN Unpack/2 -> Signal Specification/1  "VehCAN_BrkCtrl_Vehicle_speed"
  VM_Ctrl_VehCAN Unpack/1 -> Terminator4/1  "VehCAN_BrkCtrl_Regen_brake_torque_request"
  VehCAN_Msg/1 -> VM_Ctrl_VehCAN Unpack/1
  Signal Specification/1 -> BrkCtrl_Vehicle_speed/1  "BrkCtrl_Vehicle_speed"
